simulink model "Assignment1_rate_adaptive"  (R2017b)
settings: Solver=FixedStepAuto  StartTime=0.0  StopTime=inf  FixedStep=0.001  RelTol=1e-3  EnableMultiTasking=on
undefined symbols (not defined in the file): D10, D11, D12, D2, D5, D8, D9, PTA0, PTA2, PTB9, PTC4, PTD0, PTD2, PTD3, sigbuilder_block
libraries: frdmk64flib x11, dspstat3 x1
settings Model: ExtModeTrigDuration=5  Creator=montema2  LastModifiedBy=puerstee
settings OptimizationCC: PassReuseOutputArgsAs=Individual arguments  MaxStackSize=64
settings DebuggingCC: ParameterTunabilityLossMsg=error
settings HardwareCC: ProdBitPerPointer=32  ProdBitPerSizeT=32  ProdBitPerPtrDiffT=32  ProdLargestAtomicInteger=Long  ProdLargestAtomicFloat=Double  ProdWordSize=32  ProdHWDeviceType=ARM Compatible->ARM Cortex
settings SFSimCC: MATLABDynamicMemAlloc=off
settings RTWCC: SystemTargetFile=ert.tlc  HardwareBoard=NXP FRDM-K64F  TemplateMakefile=ert_default_tmf  GenerateReport=on  Toolchain=GNU Tools for ARM Embedded Processors  IncludeHyperlinkInReport=on  LaunchReport=on  GenerateTraceInfo=on  GenerateTraceReport=on  GenerateTraceReportSl=on  GenerateTraceReportSf=on  GenerateTraceReportEml=on
settings CodeAppCC: ForceParamTrailComments=on  IgnoreCustomStorageClasses=off  OperatorAnnotations=on  SimulinkDataObjDesc=on  SFDataObjDesc=on  InsertBlockDesc=on
settings ERTTargetCC: SupportContinuousTime=on

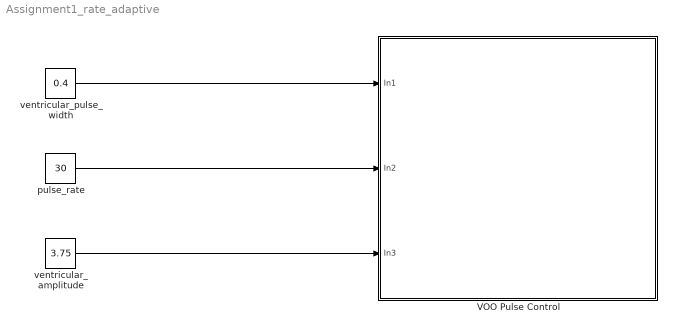
== system Assignment1_rate_adaptive ==
  VOO Pulse Control : Subsystem
  pulse_rate : Constant  Value=30  OutDataTypeStr=single
  ventricular_amplitude : Constant  Value=3.75
  ventricular_pulse_width : Constant  Value=0.4
  wires:
  ventricular_pulse_width/1 -> VOO Pulse Control/1(In1)
  pulse_rate/1 -> VOO Pulse Control/2(In2)
  ventricular_amplitude/1 -> VOO Pulse Control/3(In3)

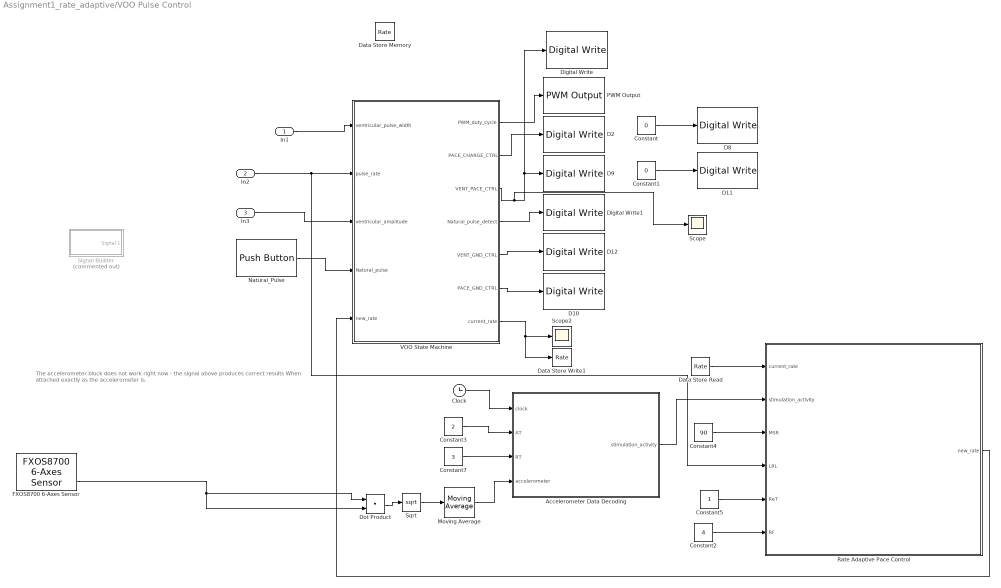
== system Assignment1_rate_adaptive/VOO Pulse Control ==
  note: The accelerometer block does not work right now - the signal above produces correct results
      | When attached exactly as the accelerometer is.
  In1 : Inport
  In2 : Inport  Port=2
  In3 : Inport  Port=3
  "Accelerometer Data Decoding " : Stateflow chart  TreatAsAtomicUnit=on
  Clock : Clock
  Constant : Constant  Value=0
  Constant1 : Constant  Value=0
  Constant2 : Constant  Value=4  OutDataTypeStr=single
  Constant3 : Constant  Value=2  OutDataTypeStr=single
  Constant4 : Constant  Value=90  OutDataTypeStr=single
  Constant5 : Constant  OutDataTypeStr=single
  Constant7 : Constant  Value=3  OutDataTypeStr=single
  D10 : frdmk64flib/Digital Write  Whichpin=PTD0 (D10)
      settings: SourceProductName=Simulink Coder Support Package for NXP FRDM-K64F Board
  D11 : frdmk64flib/Digital Write  Whichpin=PTD2 (D11)
      settings: SourceProductName=Simulink Coder Support Package for NXP FRDM-K64F Board
  D12 : frdmk64flib/Digital Write  Whichpin=PTD3 (D12)
      settings: SourceProductName=Simulink Coder Support Package for NXP FRDM-K64F Board
  D2 : frdmk64flib/Digital Write  Whichpin=PTB9 (D2)
      settings: SourceProductName=Simulink Coder Support Package for NXP FRDM-K64F Board
  D8 : frdmk64flib/Digital Write  Whichpin=PTA0 (D8)
      settings: SourceProductName=Simulink Coder Support Package for NXP FRDM-K64F Board
  D9 : frdmk64flib/Digital Write  Whichpin=PTC4 (D9)
      settings: SourceProductName=Simulink Coder Support Package for NXP FRDM-K64F Board
  Data Store Memory : DataStoreMemory  DataStoreName=Rate  ReadBeforeWriteMsg=warning  WriteAfterWriteMsg=warning  WriteAfterReadMsg=warning  ShowAdditionalParam=off  OutDataTypeStr=single
  Data Store Read : DataStoreRead  DataStoreName=Rate  DataStoreElements=Rate
  Data Store Write1 : DataStoreWrite  DataStoreName=Rate  DataStoreElements=Rate
  Digital Write : frdmk64flib/Digital Write  Whichpin=RED_LED
      settings: SourceProductName=Simulink Coder Support Package for NXP FRDM-K64F Board
  Digital Write1 : frdmk64flib/Digital Write  Whichpin=BLUE_LED
      settings: SourceProductName=Simulink Coder Support Package for NXP FRDM-K64F Board
  Dot Product : DotProduct  InputSameDT=on  OutDataTypeStr=Inherit: Inherit via internal rule
  FXOS8700 6-Axes Sensor : frdmk64flib/FXOS8700 6-Axes Sensor  Activesensor=Accelerometer and Magnetometer  ODR=800Hz  HybridODR=400Hz  Accelfullrange=-4g to +4g  SampleTime=-1
      settings: SourceProductName=Simulink Coder Support Package for NXP FRDM-K64F Board
  Moving Average : dspstat3/Moving Average  Method=Sliding window  SpecifyWindowLength=on  WindowLength=500  ForgettingFactor=0.9  SimulateUsing=Code generation
  Natural_Pulse : frdmk64flib/Push Button  Whichswitch=SW2  SampleTime1=-1
      settings: SourceProductName=Simulink Coder Support Package for NXP FRDM-K64F Board
  PWM Output : frdmk64flib/PWM Output  Whichpin=PTA2 (D5)  InitialFrequency=1000  InitialDutyCycle=0
      settings: SourceProductName=Simulink Coder Support Package for NXP FRDM-K64F Board
  "Rate Adaptive Pace Control " : Stateflow chart  TreatAsAtomicUnit=on
  Scope : Scope
  Scope2 : Scope
  Signal Builder : Subsystem  Tag=STV Subsys  Commented=on  LoadFcn=sigbuilder_block('load');  StartFcn=sigbuilder_block('start');  StopFcn=sigbuilder_block('stop');  ClipboardFcn=sigbuilder_block('clipboard');  mask(Sigbuilder block){tuvar=[0:10]}
      mask help: Simulink:masks:SigbuilderBlock_MD
      mask init:
      | if ~strcmp(get_param(bdroot(gcbh),'SimulationStatus'),'stopped') tuvar = sigbuilder_block('maskInit'); end
      settings: CopyFcn=sigbuilder_block('copy');  DeleteFcn=sigbuilder_block('delete');  ModelCloseFcn=sigbuilder_block('modelClose');  PreSaveFcn=sigbuilder_block('preSave');  PauseFcn=sigbuilder_block('pause');  ContinueFcn=sigbuilder_block('continue');  NameChangeFcn=sigbuilder_block('namechange');  OpenFcn=sigbuilder_block('open',[405 118.75 550.5 366 ]);  CloseFcn=sigbuilder_block('close');
      mask Display: plot(0, 0, 100, 100,[2, 2, 32, 32, 2], [68, 8, 8, 68, 68],[32, 2], [38, 38], [32, 19, 2],[53, 60, 44], [32, 17, 17, 2],[16, 16, 31, 31]);txt = getActiveGroup(gcbh);text(2, 100, txt,'verticalAlignment', 'top');
  Sqrt : Sqrt  SaturateOnIntegerOverflow=on
  VOO State Machine : Stateflow chart  TreatAsAtomicUnit=on
  wires:
  In1/1 -> VOO State Machine/1(ventricular_pulse_width)
  VOO State Machine/1(PWM_duty_cycle) -> PWM Output/1
  VOO State Machine/3(VENT_PACE_CTRL) -> Scope/1, Digital Write/1, D9/1
  In2/1 -> "Rate Adaptive Pace Control "/4(LRL), VOO State Machine/2(pulse_rate)
  VOO State Machine/2(PACE_CHARGE_CTRL) -> D2/1
  VOO State Machine/5(VENT_GND_CTRL) -> D12/1
  VOO State Machine/6(PACE_GND_CTRL) -> D10/1
  Constant/1 -> D8/1
  Constant1/1 -> D11/1
  Natural_Pulse/1 -> VOO State Machine/4(Natural_pulse)
  VOO State Machine/4(Natural_pulse_detect) -> Digital Write1/1
  In3/1 -> VOO State Machine/3(ventricular_amplitude)
  Moving Average/1 -> "Accelerometer Data Decoding "/4(accelerometer)
  Sqrt/1 -> Moving Average/1
  Clock/1 -> "Accelerometer Data Decoding "/1(clock)
  Constant7/1 -> "Accelerometer Data Decoding "/3(RT)
  "Accelerometer Data Decoding "/1(stimulation_activity) -> "Rate Adaptive Pace Control "/2(stimulation_activity)
  Dot Product/1 -> Sqrt/1
  Data Store Read/1 -> "Rate Adaptive Pace Control "/1(current_rate)
  Constant4/1 -> "Rate Adaptive Pace Control "/3(MSR)
  Constant3/1 -> "Accelerometer Data Decoding "/2(AT)
  Constant5/1 -> "Rate Adaptive Pace Control "/5(ReT)
  Constant2/1 -> "Rate Adaptive Pace Control "/6(RF)
  "Rate Adaptive Pace Control "/1(new_rate) -> VOO State Machine/5(new_rate)
  VOO State Machine/7(current_rate) -> Scope2/1, Data Store Write1/1
  FXOS8700 6-Axes Sensor/2 -> Dot Product/1, Dot Product/2

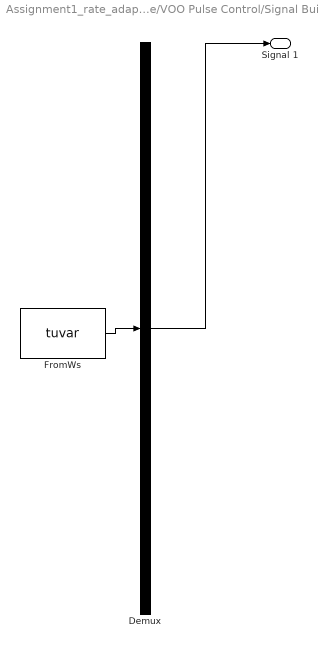
== system Assignment1_rate_adaptive/VOO Pulse Control/Signal Builder ==
  Demux : Demux  Tag=STV Demux  Outputs=1
  FromWs : FromWorkspace  Tag=STV FromWs  VariableName=tuvar  SampleTime=0
      SigBuilderData=|
      | common.afterFinalStr = 'Extrapolate'
      | common.sampleTime = 0
      | dataSet.timeRange = [0 60]
      | dataSet.name = 'Group 1'
      | sbobj.Groups.Name = 'Group 1'
      | sbobj.Groups.Signals.Name = 'Signal 1'
      | sbobj.Groups.Signals.XData = [0 0.9 13.9 19 35.1 36 58.9 60]
      | sbobj.Groups.Signals.YData = [3.02 3.02 3 0.46 0.5 3 3.02 2.01]
      | sbobj.Groups.TimeRange = [0 60]
  Signal 1 : Outport  Tag=STV Outport
  wires:
  Demux/1 -> Signal 1/1
  FromWs/1 -> Demux/1

== stateflow chart Assignment1_rate_adaptive/VOO Pulse Control/Rate Adaptive Pace Control  ==
  state const_LRL
    entry: new_rate=LRL;
  state increasing_rate
  state decreasing_rate
  state const_MSR
    entry: new_rate=MSR;
  (default) -> const_LRL : {new_rate=LRL}
  decreasing_rate -> const_LRL [order 2] : [after((1000),msec) && current_rate + (LRL-MSR)/(60*ReT) <= LRL]
  const_LRL -> increasing_rate : [stimulation_activity==true]
  increasing_rate -> decreasing_rate [order 1] : [stimulation_activity==false]
  increasing_rate -> increasing_rate [order 3] : [(current_rate+ (MSR/LRL)*RF)<MSR && after((1000),msec)]
      | {new_rate=current_rate + (MSR/LRL)*RF}
  decreasing_rate -> decreasing_rate [order 3] : [after((1000),msec) && current_rate + (LRL-MSR)/(60*ReT) > LRL]
      | {new_rate=current_rate + (LRL-MSR)/(60*ReT)}
  decreasing_rate -> increasing_rate [order 1] : [stimulation_activity==true]
  const_MSR -> decreasing_rate : [stimulation_activity==false]
  increasing_rate -> const_MSR [order 2] : [(current_rate+ (MSR/LRL)*RF) >= MSR && after((1000),msec)]
  data: new_rate output single; current_rate input single; stimulation_activity input boolean; MSR input single; LRL input single; ReT input single; RF input single

== stateflow chart Assignment1_rate_adaptive/VOO Pulse Control/Accelerometer Data Decoding  ==
  state false_state
    entry:
    stimulation_activity = false;
  state Compare_State
    entry:
    compare = clock - time;
  state true_state
    entry: stimulation_activity = true;
  (default) -> false_state
  true_state -> false_state : [accelerometer<AT]
  Compare_State -> false_state [order 1] : [accelerometer<AT]
  false_state -> Compare_State : [accelerometer>=AT]{time=clock}
  Compare_State -> Compare_State [order 2] : [compare<RT]
  Compare_State -> true_state [order 3] : [compare>=RT]
  data: clock input; stimulation_activity output boolean; AT input single; RT input single; accelerometer input double; time local; compare local

== stateflow chart Assignment1_rate_adaptive/VOO Pulse Control/VOO State Machine ==
  note: Switch States:
      | true=closed
      | false=open
  state start_state
    entry:VENT_PACE_CTRL=false;
    VENT_GND_CTRL=true;
    PACE_CHARGE_CTRL=true;
    PACE_GND_CTRL=true;
    PWM_duty_cycle=((ventricular_amplitude/5)*100);
    current_rate = pulse_rate;
  state current_into_heart
    entry:
    PACE_CHARGE_CTRL=false;
    VENT_GND_CTRL=false;
    VENT_PACE_CTRL=true;
    current_rate=new_rate;
  state current_out_of_heart
    entry:
    VENT_PACE_CTRL=false;
    PACE_CHARGE_CTRL=true;
    VENT_GND_CTRL=true;
    current_rate=new_rate;
  state natural_pace
    entry: Natural_pulse_detect=true;
    exit: Natural_pulse_detect=false;
  (default) -> start_state
  start_state -> current_into_heart [order 1] : [after(((60/current_rate)*1000),msec)]
  current_into_heart -> natural_pace [order 2] : [Natural_pulse==true]
  start_state -> natural_pace [order 2] : [Natural_pulse==true]
  natural_pace -> start_state : [Natural_pulse==false]
  current_into_heart -> current_out_of_heart [order 1] : [after((ventricular_pulse_width),msec)]
  current_out_of_heart -> current_into_heart [order 1] : [after(((60/current_rate)*1000)-(ventricular_pulse_width),msec)]
  current_out_of_heart -> natural_pace [order 2] : [Natural_pulse==true]
  data: ventricular_pulse_width input double; pulse_rate input single; ventricular_amplitude input double; PWM_duty_cycle output double [0..100]; PACE_CHARGE_CTRL output boolean; VENT_PACE_CTRL output boolean; Natural_pulse_detect output; VENT_GND_CTRL output boolean; PACE_GND_CTRL output boolean; Natural_pulse input boolean; new_rate input single; current_rate output single
